simulink model "wheel_leg"  (R2024b)
settings: Solver=FixedStepAuto  StartTime=0.0  StopTime=10  FixedStep=0.001  RelTol=1e-3  AbsTol=1e-3  EnableMultiTasking=on
model workspace: external: MATLAB File UseBodyVel.m (data not in the file)
values from neighbouring files (symbols this model uses):
  g = 9.81    [LQR_calc.m]    (also in UseBodyVel.m)
  joint_distance = 0.11    [LQR_calc.m]    (also in UseBodyVel.m)
  l = -0.014    [LQR_calc.m]    (also in UseBodyVel.m)
  l_active_leg = 0.14    [LQR_calc.m]    (also in UseBodyVel.m)
  l_slave_leg = 0.24    [LQR_calc.m]    (also in UseBodyVel.m)
  M = 12    [LQR_calc.m]    (also in UseBodyVel.m)
  m_active_leg = 0.174    [LQR_calc.m]    (also in UseBodyVel.m)
  m_slave_leg = 0.180    (= 0.18)    [LQR_calc.m]    (also in UseBodyVel.m)
  mw = 0.58    [LQR_calc.m]    (also in UseBodyVel.m)
  N = mp*(x_ddot+L*theta_ddot*cos(theta)-L*theta_dot^2*sin(theta))+N_M    [UseBodyVel.m]
  X = [theta,theta_dot,x,x_dot,phi,phi_dot].'    [UseBodyVel.m]
undefined symbols (not defined in the file or in its folder): Y, Z
libraries: sm_lib x65, nesl_utility x25, dspfdesign x3
(part 3 of 3)

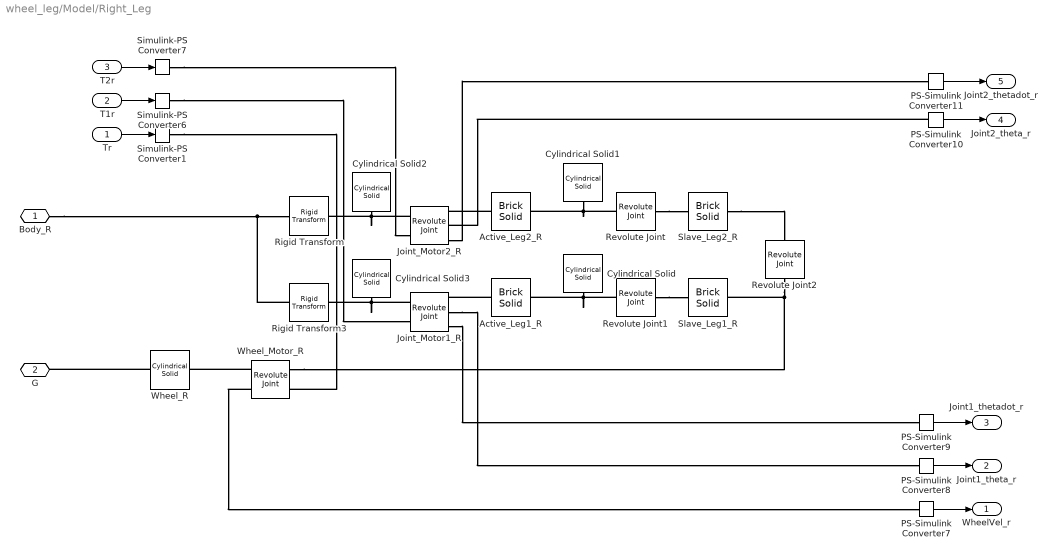
== system wheel_leg/Model/Right_Leg ==
  Tr : Inport
  T1r : Inport  Port=2
  T2r : Inport  Port=3
  Active_Leg1_R : sm_lib/Body Elements/Brick Solid  BrickDimensions=[0.02 l_active_leg 0.01]  BrickDimensionsUnits=m  ExportEntireGeometry=off  InertiaType=CalculateFromGeometry  BasedOnType=Mass  Density=1000  DensityUnits=kg/m^3  Mass=m_active_leg  MassUnits=kg  CenterOfMass=[0 0 0]  CenterOfMassUnits=m  MomentsOfInertia=[1 1 1]  MomentsOfInertiaUnits=kg*m^2  ProductsOfInertia=[0 0 0]  ProductsOfInertiaUnits=kg*m^2  GraphicType=FromGeometry  MarkerShape=Sphere  MarkerSize=10  GraphicVisPropType=SimpleVisualProperties  GraphicDiffuseColor=[0.5 0.5 0.5]  GraphicOpacity=1.0  GraphicSpecularColor=[0.5 0.5 0.5 1.0]  GraphicAmbientColor=[0.15 0.15 0.15 1.0]  GraphicEmissiveColor=[0.0 0.0 0.0 1.0]  GraphicShininess=75  DoExposeReferenceFrame=off  SerializedFrames=<Frames><Frame><Id>Frame1</Id><Value><Name>T</Name><Origin><Source>GeometricFeature</Source><FeatureName>+y surface</FeatureName></Origin><PrimaryAxis><DefinedDirection>+Z</DefinedDirection><Source>ReferenceFrame</Source><SourceDirection>+Z</SourceDirection><FeatureName></FeatureName></PrimaryAxis><SecondaryAxis><DefinedDirection>+X</DefinedDirection><Source>ReferenceFrame</Source><SourceDirection>+X</SourceDirection><FeatureName></FeatureName></SecondaryAxis></Value></Frame><Frame><Id>Frame2</Id><Value><Name>B</Name><Origin><Source>GeometricFeature</Source><FeatureName>-y surface</FeatureName></Origin><PrimaryAxis><DefinedDirection>+Z</DefinedDirection><Source>ReferenceFrame</Source><SourceDirection>+Z</SourceDirection><FeatureName></FeatureName></PrimaryAxis><SecondaryAxis><DefinedDirection>+X</DefinedDirection><Source>ReferenceFrame</Source><SourceDirection>+X</SourceDirection><FeatureName></FeatureName></SecondaryAxis></Value></Frame></Frames>
  Active_Leg2_R : sm_lib/Body Elements/Brick Solid  BrickDimensions=[0.02 l_active_leg 0.01]  BrickDimensionsUnits=m  ExportEntireGeometry=off  InertiaType=CalculateFromGeometry  BasedOnType=Mass  Density=1000  DensityUnits=kg/m^3  Mass=m_active_leg  MassUnits=kg  CenterOfMass=[0 0 0]  CenterOfMassUnits=m  MomentsOfInertia=[1 1 1]  MomentsOfInertiaUnits=kg*m^2  ProductsOfInertia=[0 0 0]  ProductsOfInertiaUnits=kg*m^2  GraphicType=FromGeometry  MarkerShape=Sphere  MarkerSize=10  GraphicVisPropType=SimpleVisualProperties  GraphicDiffuseColor=[0.5 0.5 0.5]  GraphicOpacity=1.0  GraphicSpecularColor=[0.5 0.5 0.5 1.0]  GraphicAmbientColor=[0.15 0.15 0.15 1.0]  GraphicEmissiveColor=[0.0 0.0 0.0 1.0]  GraphicShininess=75  DoExposeReferenceFrame=off  SerializedFrames=<Frames><Frame><Id>Frame1</Id><Value><Name>T</Name><Origin><Source>GeometricFeature</Source><FeatureName>+y surface</FeatureName></Origin><PrimaryAxis><DefinedDirection>+Z</DefinedDirection><Source>ReferenceFrame</Source><SourceDirection>+Z</SourceDirection><FeatureName></FeatureName></PrimaryAxis><SecondaryAxis><DefinedDirection>+X</DefinedDirection><Source>ReferenceFrame</Source><SourceDirection>+X</SourceDirection><FeatureName></FeatureName></SecondaryAxis></Value></Frame><Frame><Id>Frame2</Id><Value><Name>B</Name><Origin><Source>GeometricFeature</Source><FeatureName>-y surface</FeatureName></Origin><PrimaryAxis><DefinedDirection>+Z</DefinedDirection><Source>ReferenceFrame</Source><SourceDirection>+Z</SourceDirection><FeatureName></FeatureName></PrimaryAxis><SecondaryAxis><DefinedDirection>+X</DefinedDirection><Source>ReferenceFrame</Source><SourceDirection>+X</SourceDirection><FeatureName></FeatureName></SecondaryAxis></Value></Frame></Frames>
  Cylindrical Solid : sm_lib/Body Elements/Cylindrical Solid  CylinderRadius=0.01  CylinderRadiusUnits=m  CylinderLength=0.03  CylinderLengthUnits=m  ExportEntireGeometry=off  InertiaType=CalculateFromGeometry  BasedOnType=Mass  Density=1000  DensityUnits=kg/m^3  Mass=0  MassUnits=kg  CenterOfMass=[0 0 0]  CenterOfMassUnits=m  MomentsOfInertia=[1 1 1]  MomentsOfInertiaUnits=kg*m^2  ProductsOfInertia=[0 0 0]  ProductsOfInertiaUnits=kg*m^2  GraphicType=FromGeometry  MarkerShape=Sphere  MarkerSize=10  GraphicVisPropType=SimpleVisualProperties  GraphicDiffuseColor=[0 1 0]  GraphicOpacity=1.0  GraphicSpecularColor=[0.5 0.5 0.5 1.0]  GraphicAmbientColor=[0.15 0.15 0.15 1.0]  GraphicEmissiveColor=[0.0 0.0 0.0 1.0]  GraphicShininess=75  DoExposeReferenceFrame=on  SerializedFrames=<Frames/>
  Cylindrical Solid1 : sm_lib/Body Elements/Cylindrical Solid  CylinderRadius=0.01  CylinderRadiusUnits=m  CylinderLength=0.03  CylinderLengthUnits=m  ExportEntireGeometry=off  InertiaType=CalculateFromGeometry  BasedOnType=Mass  Density=1000  DensityUnits=kg/m^3  Mass=0  MassUnits=kg  CenterOfMass=[0 0 0]  CenterOfMassUnits=m  MomentsOfInertia=[1 1 1]  MomentsOfInertiaUnits=kg*m^2  ProductsOfInertia=[0 0 0]  ProductsOfInertiaUnits=kg*m^2  GraphicType=FromGeometry  MarkerShape=Sphere  MarkerSize=10  GraphicVisPropType=SimpleVisualProperties  GraphicDiffuseColor=[0 1 0]  GraphicOpacity=1.0  GraphicSpecularColor=[0.5 0.5 0.5 1.0]  GraphicAmbientColor=[0.15 0.15 0.15 1.0]  GraphicEmissiveColor=[0.0 0.0 0.0 1.0]  GraphicShininess=75  DoExposeReferenceFrame=on  SerializedFrames=<Frames/>
  Cylindrical Solid2 : sm_lib/Body Elements/Cylindrical Solid  CylinderRadius=0.02  CylinderRadiusUnits=m  CylinderLength=0.02  CylinderLengthUnits=m  ExportEntireGeometry=off  InertiaType=CalculateFromGeometry  BasedOnType=Mass  Density=1000  DensityUnits=kg/m^3  Mass=0  MassUnits=kg  CenterOfMass=[0 0 0]  CenterOfMassUnits=m  MomentsOfInertia=[1 1 1]  MomentsOfInertiaUnits=kg*m^2  ProductsOfInertia=[0 0 0]  ProductsOfInertiaUnits=kg*m^2  GraphicType=FromGeometry  MarkerShape=Sphere  MarkerSize=10  GraphicVisPropType=SimpleVisualProperties  GraphicDiffuseColor=[1.0 0.6 0.6]  GraphicOpacity=1.0  GraphicSpecularColor=[0.5 0.5 0.5 1.0]  GraphicAmbientColor=[0.15 0.15 0.15 1.0]  GraphicEmissiveColor=[0.0 0.0 0.0 1.0]  GraphicShininess=75  DoExposeReferenceFrame=on  SerializedFrames=<Frames/>
  Cylindrical Solid3 : sm_lib/Body Elements/Cylindrical Solid  CylinderRadius=0.02  CylinderRadiusUnits=m  CylinderLength=0.02  CylinderLengthUnits=m  ExportEntireGeometry=off  InertiaType=CalculateFromGeometry  BasedOnType=Mass  Density=1000  DensityUnits=kg/m^3  Mass=0  MassUnits=kg  CenterOfMass=[0 0 0]  CenterOfMassUnits=m  MomentsOfInertia=[1 1 1]  MomentsOfInertiaUnits=kg*m^2  ProductsOfInertia=[0 0 0]  ProductsOfInertiaUnits=kg*m^2  GraphicType=FromGeometry  MarkerShape=Sphere  MarkerSize=10  GraphicVisPropType=SimpleVisualProperties  GraphicDiffuseColor=[1.0 0.6 0.6]  GraphicOpacity=1.0  GraphicSpecularColor=[0.5 0.5 0.5 1.0]  GraphicAmbientColor=[0.15 0.15 0.15 1.0]  GraphicEmissiveColor=[0.0 0.0 0.0 1.0]  GraphicShininess=75  DoExposeReferenceFrame=on  SerializedFrames=<Frames/>
  Joint_Motor1_R : sm_lib/Joints/Revolute Joint  JointMode=Normal  CompositeWrenchDir=FollowerOnBase  CompositeWrenchFrame=BaseFrame  SenseConstraintForce=off  SenseConstraintTorque=off  SenseTotalForce=off  SenseTotalTorque=off  PositionTargetSpecify=on  PositionTargetPriority=High  PositionTargetValue=-50  PositionTargetValueUnits=deg  VelocityTargetSpecify=off  VelocityTargetPriority=High  VelocityTargetValue=0  VelocityTargetValueUnits=deg/s  EquilibriumPosition=0  EquilibriumPositionUnits=deg  SpringStiffness=0  SpringStiffnessUnits=N*m/deg  DampingCoefficient=0  DampingCoefficientUnits=N*m/(deg/s)  LowerLimitSpecify=off  LowerLimitBound=-100  LowerLimitBoundUnits=deg  LowerLimitStiffness=1e4  LowerLimitStiffnessUnits=N*m/deg  LowerLimitDamping=10  LowerLimitDampingUnits=N*m/(deg/s)  LowerLimitTransitionRegionWidth=0.1  LowerLimitTransitionRegionWidthUnits=deg  UpperLimitSpecify=off  UpperLimitBound=50  UpperLimitBoundUnits=deg  UpperLimitStiffness=1e4  UpperLimitStiffnessUnits=N*m/deg  UpperLimitDamping=10  UpperLimitDampingUnits=N*m/(deg/s)  UpperLimitTransitionRegionWidth=0.1  UpperLimitTransitionRegionWidthUnits=deg  TorqueActuationMode=InputTorque  MotionActuationMode=ComputedMotion  SensePosition=on  SenseVelocity=on  SenseAcceleration=off  SenseTorqueForce=off  SenseLowerLimitTorqueForce=off  SenseUpperLimitTorqueForce=off
  Joint_Motor2_R : sm_lib/Joints/Revolute Joint  JointMode=Normal  CompositeWrenchDir=FollowerOnBase  CompositeWrenchFrame=BaseFrame  SenseConstraintForce=off  SenseConstraintTorque=off  SenseTotalForce=off  SenseTotalTorque=off  PositionTargetSpecify=on  PositionTargetPriority=High  PositionTargetValue=50  PositionTargetValueUnits=deg  VelocityTargetSpecify=off  VelocityTargetPriority=High  VelocityTargetValue=0  VelocityTargetValueUnits=deg/s  EquilibriumPosition=0  EquilibriumPositionUnits=deg  SpringStiffness=0  SpringStiffnessUnits=N*m/deg  DampingCoefficient=0  DampingCoefficientUnits=N*m/(deg/s)  LowerLimitSpecify=off  LowerLimitBound=10  LowerLimitBoundUnits=deg  LowerLimitStiffness=1e4  LowerLimitStiffnessUnits=N*m/deg  LowerLimitDamping=10  LowerLimitDampingUnits=N*m/(deg/s)  LowerLimitTransitionRegionWidth=0.1  LowerLimitTransitionRegionWidthUnits=deg  UpperLimitSpecify=off  UpperLimitBound=100  UpperLimitBoundUnits=deg  UpperLimitStiffness=1e4  UpperLimitStiffnessUnits=N*m/deg  UpperLimitDamping=10  UpperLimitDampingUnits=N*m/(deg/s)  UpperLimitTransitionRegionWidth=0.1  UpperLimitTransitionRegionWidthUnits=deg  TorqueActuationMode=InputTorque  MotionActuationMode=ComputedMotion  SensePosition=on  SenseVelocity=on  SenseAcceleration=off  SenseTorqueForce=off  SenseLowerLimitTorqueForce=off  SenseUpperLimitTorqueForce=off
  PS-Simulink Converter10 : nesl_utility/PS-Simulink Converter  PhysicalDomain=network_engine_domain  SubClassName=ps_output  LeftPortType=input  RightPortType=output  PseudoPeriodic=off  Frequencies=[]  VectorFormat=inherit  Unit=rad  AffineConversion=off
  PS-Simulink Converter11 : nesl_utility/PS-Simulink Converter  PhysicalDomain=network_engine_domain  SubClassName=ps_output  LeftPortType=input  RightPortType=output  PseudoPeriodic=off  Frequencies=[]  VectorFormat=inherit  Unit=rad/s  AffineConversion=off
  PS-Simulink Converter7 : nesl_utility/PS-Simulink Converter  PhysicalDomain=network_engine_domain  SubClassName=ps_output  LeftPortType=input  RightPortType=output  PseudoPeriodic=off  Frequencies=[]  VectorFormat=inherit  Unit=rad/s  AffineConversion=off
  PS-Simulink Converter8 : nesl_utility/PS-Simulink Converter  PhysicalDomain=network_engine_domain  SubClassName=ps_output  LeftPortType=input  RightPortType=output  PseudoPeriodic=off  Frequencies=[]  VectorFormat=inherit  Unit=rad  AffineConversion=off
  PS-Simulink Converter9 : nesl_utility/PS-Simulink Converter  PhysicalDomain=network_engine_domain  SubClassName=ps_output  LeftPortType=input  RightPortType=output  PseudoPeriodic=off  Frequencies=[]  VectorFormat=inherit  Unit=rad/s  AffineConversion=off
  Revolute Joint : sm_lib/Joints/Revolute Joint  JointMode=Normal  CompositeWrenchDir=FollowerOnBase  CompositeWrenchFrame=BaseFrame  SenseConstraintForce=off  SenseConstraintTorque=off  SenseTotalForce=off  SenseTotalTorque=off  PositionTargetSpecify=off  PositionTargetPriority=High  PositionTargetValue=0  PositionTargetValueUnits=deg  VelocityTargetSpecify=off  VelocityTargetPriority=High  VelocityTargetValue=0  VelocityTargetValueUnits=deg/s  EquilibriumPosition=0  EquilibriumPositionUnits=deg  SpringStiffness=0  SpringStiffnessUnits=N*m/deg  DampingCoefficient=0  DampingCoefficientUnits=N*m/(deg/s)  LowerLimitSpecify=off  LowerLimitBound=-90  LowerLimitBoundUnits=deg  LowerLimitStiffness=1e4  LowerLimitStiffnessUnits=N*m/deg  LowerLimitDamping=10  LowerLimitDampingUnits=N*m/(deg/s)  LowerLimitTransitionRegionWidth=0.1  LowerLimitTransitionRegionWidthUnits=deg  UpperLimitSpecify=off  UpperLimitBound=90  UpperLimitBoundUnits=deg  UpperLimitStiffness=1e4  UpperLimitStiffnessUnits=N*m/deg  UpperLimitDamping=10  UpperLimitDampingUnits=N*m/(deg/s)  UpperLimitTransitionRegionWidth=0.1  UpperLimitTransitionRegionWidthUnits=deg  TorqueActuationMode=NoTorque  MotionActuationMode=ComputedMotion  SensePosition=off  SenseVelocity=off  SenseAcceleration=off  SenseTorqueForce=off  SenseLowerLimitTorqueForce=off  SenseUpperLimitTorqueForce=off
  Revolute Joint1 : sm_lib/Joints/Revolute Joint  JointMode=Normal  CompositeWrenchDir=FollowerOnBase  CompositeWrenchFrame=BaseFrame  SenseConstraintForce=off  SenseConstraintTorque=off  SenseTotalForce=off  SenseTotalTorque=off  PositionTargetSpecify=off  PositionTargetPriority=High  PositionTargetValue=0  PositionTargetValueUnits=deg  VelocityTargetSpecify=off  VelocityTargetPriority=High  VelocityTargetValue=0  VelocityTargetValueUnits=deg/s  EquilibriumPosition=0  EquilibriumPositionUnits=deg  SpringStiffness=0  SpringStiffnessUnits=N*m/deg  DampingCoefficient=0  DampingCoefficientUnits=N*m/(deg/s)  LowerLimitSpecify=off  LowerLimitBound=-90  LowerLimitBoundUnits=deg  LowerLimitStiffness=1e4  LowerLimitStiffnessUnits=N*m/deg  LowerLimitDamping=10  LowerLimitDampingUnits=N*m/(deg/s)  LowerLimitTransitionRegionWidth=0.1  LowerLimitTransitionRegionWidthUnits=deg  UpperLimitSpecify=off  UpperLimitBound=90  UpperLimitBoundUnits=deg  UpperLimitStiffness=1e4  UpperLimitStiffnessUnits=N*m/deg  UpperLimitDamping=10  UpperLimitDampingUnits=N*m/(deg/s)  UpperLimitTransitionRegionWidth=0.1  UpperLimitTransitionRegionWidthUnits=deg  TorqueActuationMode=NoTorque  MotionActuationMode=ComputedMotion  SensePosition=off  SenseVelocity=off  SenseAcceleration=off  SenseTorqueForce=off  SenseLowerLimitTorqueForce=off  SenseUpperLimitTorqueForce=off
  Revolute Joint2 : sm_lib/Joints/Revolute Joint  JointMode=Normal  CompositeWrenchDir=FollowerOnBase  CompositeWrenchFrame=BaseFrame  SenseConstraintForce=off  SenseConstraintTorque=off  SenseTotalForce=off  SenseTotalTorque=off  PositionTargetSpecify=off  PositionTargetPriority=High  PositionTargetValue=0  PositionTargetValueUnits=deg  VelocityTargetSpecify=off  VelocityTargetPriority=High  VelocityTargetValue=0  VelocityTargetValueUnits=deg/s  EquilibriumPosition=0  EquilibriumPositionUnits=deg  SpringStiffness=0  SpringStiffnessUnits=N*m/deg  DampingCoefficient=0  DampingCoefficientUnits=N*m/(deg/s)  LowerLimitSpecify=off  LowerLimitBound=-90  LowerLimitBoundUnits=deg  LowerLimitStiffness=1e4  LowerLimitStiffnessUnits=N*m/deg  LowerLimitDamping=10  LowerLimitDampingUnits=N*m/(deg/s)  LowerLimitTransitionRegionWidth=0.1  LowerLimitTransitionRegionWidthUnits=deg  UpperLimitSpecify=off  UpperLimitBound=90  UpperLimitBoundUnits=deg  UpperLimitStiffness=1e4  UpperLimitStiffnessUnits=N*m/deg  UpperLimitDamping=10  UpperLimitDampingUnits=N*m/(deg/s)  UpperLimitTransitionRegionWidth=0.1  UpperLimitTransitionRegionWidthUnits=deg  TorqueActuationMode=NoTorque  MotionActuationMode=ComputedMotion  SensePosition=off  SenseVelocity=off  SenseAcceleration=off  SenseTorqueForce=off  SenseLowerLimitTorqueForce=off  SenseUpperLimitTorqueForce=off
  Rigid Transform : sm_lib/Frames and Transforms/Rigid Transform  RotationMethod=None  FollAlignAxisA=+X  BaseAlignAxisA=+Y  FollAlignAxisB=+Y  BaseAlignAxisB=+Z  RotationStandardAxis=+Z  RotationAngle=0.0  RotationAngleUnits=deg  RotationArbitraryAxis=[0 0 1]  RotationSequenceAxes=FollowerAxes  RotationSequence=XYX  RotationSequenceAngles=[0 0 0]  RotationSequenceAnglesUnits=deg  RotationMatrix=[1 0 0; 0 1 0; 0 0 1]  Quaternion=[1 0 0 0]  TranslationMethod=Cartesian  TranslationCartesianOffset=[joint_distance/2 -l 0]  TranslationCartesianOffsetUnits=m  TranslationStandardAxis=+Z  TranslationStandardOffset=0  TranslationStandardOffsetUnits=m  TranslationROffset=0  TranslationROffsetUnits=m  TranslationThetaOffset=0  TranslationThetaOffsetUnits=deg  TranslationZOffset=0  TranslationZOffsetUnits=m
  Rigid Transform3 : sm_lib/Frames and Transforms/Rigid Transform  RotationMethod=None  FollAlignAxisA=+X  BaseAlignAxisA=+Y  FollAlignAxisB=+Y  BaseAlignAxisB=+Z  RotationStandardAxis=+Z  RotationAngle=0.0  RotationAngleUnits=deg  RotationArbitraryAxis=[0 0 1]  RotationSequenceAxes=FollowerAxes  RotationSequence=XYX  RotationSequenceAngles=[0 0 0]  RotationSequenceAnglesUnits=deg  RotationMatrix=[1 0 0; 0 1 0; 0 0 1]  Quaternion=[1 0 0 0]  TranslationMethod=Cartesian  TranslationCartesianOffset=[-joint_distance/2 -l 0]  TranslationCartesianOffsetUnits=m  TranslationStandardAxis=+Z  TranslationStandardOffset=0  TranslationStandardOffsetUnits=m  TranslationROffset=0  TranslationROffsetUnits=m  TranslationThetaOffset=0  TranslationThetaOffsetUnits=deg  TranslationZOffset=0  TranslationZOffsetUnits=m
  Simulink-PS Converter1 : nesl_utility/Simulink-PS Converter  PhysicalDomain=network_engine_domain  SubClassName=ps_input  LeftPortType=input  RightPortType=output  PseudoPeriodic=off  Frequencies=[]  NoiseDistribution=none  NoiseParameters=[]  Unit=N*m  AffineConversion=off  FilteringAndDerivatives=provide  SimscapeFilterOrder=1  InputFilterTimeConstant=0.001  UdotUserProvided=0
  Simulink-PS Converter6 : nesl_utility/Simulink-PS Converter  PhysicalDomain=network_engine_domain  SubClassName=ps_input  LeftPortType=input  RightPortType=output  PseudoPeriodic=off  Frequencies=[]  NoiseDistribution=none  NoiseParameters=[]  Unit=N*m  AffineConversion=off  FilteringAndDerivatives=provide  SimscapeFilterOrder=1  InputFilterTimeConstant=0.001  UdotUserProvided=0
  Simulink-PS Converter7 : nesl_utility/Simulink-PS Converter  PhysicalDomain=network_engine_domain  SubClassName=ps_input  LeftPortType=input  RightPortType=output  PseudoPeriodic=off  Frequencies=[]  NoiseDistribution=none  NoiseParameters=[]  Unit=N*m  AffineConversion=off  FilteringAndDerivatives=provide  SimscapeFilterOrder=1  InputFilterTimeConstant=0.001  UdotUserProvided=0
  Slave_Leg1_R : sm_lib/Body Elements/Brick Solid  BrickDimensions=[0.02 l_slave_leg 0.01]  BrickDimensionsUnits=m  ExportEntireGeometry=off  InertiaType=CalculateFromGeometry  BasedOnType=Mass  Density=1000  DensityUnits=kg/m^3  Mass=m_slave_leg  MassUnits=kg  CenterOfMass=[0 0 0]  CenterOfMassUnits=m  MomentsOfInertia=[1 1 1]  MomentsOfInertiaUnits=kg*m^2  ProductsOfInertia=[0 0 0]  ProductsOfInertiaUnits=kg*m^2  GraphicType=FromGeometry  MarkerShape=Sphere  MarkerSize=10  GraphicVisPropType=SimpleVisualProperties  GraphicDiffuseColor=[0.5 0.5 0.5]  GraphicOpacity=1.0  GraphicSpecularColor=[0.5 0.5 0.5 1.0]  GraphicAmbientColor=[0.15 0.15 0.15 1.0]  GraphicEmissiveColor=[0.0 0.0 0.0 1.0]  GraphicShininess=75  DoExposeReferenceFrame=off  SerializedFrames=<Frames><Frame><Id>Frame1</Id><Value><Name>T</Name><Origin><Source>GeometricFeature</Source><FeatureName>+y surface</FeatureName></Origin><PrimaryAxis><DefinedDirection>+Z</DefinedDirection><Source>ReferenceFrame</Source><SourceDirection>+Z</SourceDirection><FeatureName></FeatureName></PrimaryAxis><SecondaryAxis><DefinedDirection>+X</DefinedDirection><Source>ReferenceFrame</Source><SourceDirection>+X</SourceDirection><FeatureName></FeatureName></SecondaryAxis></Value></Frame><Frame><Id>Frame2</Id><Value><Name>B</Name><Origin><Source>GeometricFeature</Source><FeatureName>-y surface</FeatureName></Origin><PrimaryAxis><DefinedDirection>+Z</DefinedDirection><Source>ReferenceFrame</Source><SourceDirection>+Z</SourceDirection><FeatureName></FeatureName></PrimaryAxis><SecondaryAxis><DefinedDirection>+X</DefinedDirection><Source>ReferenceFrame</Source><SourceDirection>+X</SourceDirection><FeatureName></FeatureName></SecondaryAxis></Value></Frame></Frames>
  Slave_Leg2_R : sm_lib/Body Elements/Brick Solid  BrickDimensions=[0.02 l_slave_leg 0.01]  BrickDimensionsUnits=m  ExportEntireGeometry=off  InertiaType=CalculateFromGeometry  BasedOnType=Mass  Density=1000  DensityUnits=kg/m^3  Mass=m_slave_leg  MassUnits=kg  CenterOfMass=[0 0 0]  CenterOfMassUnits=m  MomentsOfInertia=[1 1 1]  MomentsOfInertiaUnits=kg*m^2  ProductsOfInertia=[0 0 0]  ProductsOfInertiaUnits=kg*m^2  GraphicType=FromGeometry  MarkerShape=Sphere  MarkerSize=10  GraphicVisPropType=SimpleVisualProperties  GraphicDiffuseColor=[0.5 0.5 0.5]  GraphicOpacity=1.0  GraphicSpecularColor=[0.5 0.5 0.5 1.0]  GraphicAmbientColor=[0.15 0.15 0.15 1.0]  GraphicEmissiveColor=[0.0 0.0 0.0 1.0]  GraphicShininess=75  DoExposeReferenceFrame=off  SerializedFrames=<Frames><Frame><Id>Frame1</Id><Value><Name>T</Name><Origin><Source>GeometricFeature</Source><FeatureName>+y surface</FeatureName></Origin><PrimaryAxis><DefinedDirection>+Z</DefinedDirection><Source>ReferenceFrame</Source><SourceDirection>+Z</SourceDirection><FeatureName></FeatureName></PrimaryAxis><SecondaryAxis><DefinedDirection>+X</DefinedDirection><Source>ReferenceFrame</Source><SourceDirection>+X</SourceDirection><FeatureName></FeatureName></SecondaryAxis></Value></Frame><Frame><Id>Frame2</Id><Value><Name>B</Name><Origin><Source>GeometricFeature</Source><FeatureName>-y surface</FeatureName></Origin><PrimaryAxis><DefinedDirection>+Z</DefinedDirection><Source>ReferenceFrame</Source><SourceDirection>+Z</SourceDirection><FeatureName></FeatureName></PrimaryAxis><SecondaryAxis><DefinedDirection>+X</DefinedDirection><Source>ReferenceFrame</Source><SourceDirection>+X</SourceDirection><FeatureName></FeatureName></SecondaryAxis></Value></Frame></Frames>
  Wheel_Motor_R : sm_lib/Joints/Revolute Joint  JointMode=Normal  CompositeWrenchDir=FollowerOnBase  CompositeWrenchFrame=BaseFrame  SenseConstraintForce=off  SenseConstraintTorque=off  SenseTotalForce=off  SenseTotalTorque=off  PositionTargetSpecify=off  PositionTargetPriority=High  PositionTargetValue=0  PositionTargetValueUnits=deg  VelocityTargetSpecify=off  VelocityTargetPriority=High  VelocityTargetValue=0  VelocityTargetValueUnits=deg/s  EquilibriumPosition=0  EquilibriumPositionUnits=deg  SpringStiffness=0  SpringStiffnessUnits=N*m/deg  DampingCoefficient=0  DampingCoefficientUnits=N*m/(deg/s)  LowerLimitSpecify=off  LowerLimitBound=-90  LowerLimitBoundUnits=deg  LowerLimitStiffness=1e4  LowerLimitStiffnessUnits=N*m/deg  LowerLimitDamping=10  LowerLimitDampingUnits=N*m/(deg/s)  LowerLimitTransitionRegionWidth=0.1  LowerLimitTransitionRegionWidthUnits=deg  UpperLimitSpecify=off  UpperLimitBound=90  UpperLimitBoundUnits=deg  UpperLimitStiffness=1e4  UpperLimitStiffnessUnits=N*m/deg  UpperLimitDamping=10  UpperLimitDampingUnits=N*m/(deg/s)  UpperLimitTransitionRegionWidth=0.1  UpperLimitTransitionRegionWidthUnits=deg  TorqueActuationMode=InputTorque  MotionActuationMode=ComputedMotion  SensePosition=off  SenseVelocity=on  SenseAcceleration=off  SenseTorqueForce=off  SenseLowerLimitTorqueForce=off  SenseUpperLimitTorqueForce=off
  Wheel_R : sm_lib/Body Elements/Cylindrical Solid  CylinderRadius=R  CylinderRadiusUnits=m  CylinderLength=0.03  CylinderLengthUnits=m  ExportEntireGeometry=on  InertiaType=CalculateFromGeometry  BasedOnType=Mass  Density=1000  DensityUnits=kg/m^3  Mass=mw  MassUnits=kg  CenterOfMass=[0 0 0]  CenterOfMassUnits=m  MomentsOfInertia=[1 1 1]  MomentsOfInertiaUnits=kg*m^2  ProductsOfInertia=[0 0 0]  ProductsOfInertiaUnits=kg*m^2  GraphicType=FromGeometry  MarkerShape=Sphere  MarkerSize=10  GraphicVisPropType=SimpleVisualProperties  GraphicDiffuseColor=[1.0 0.2 0.2]  GraphicOpacity=1.0  GraphicSpecularColor=[0.5 0.5 0.5 1.0]  GraphicAmbientColor=[0.15 0.15 0.15 1.0]  GraphicEmissiveColor=[0.0 0.0 0.0 1.0]  GraphicShininess=75  DoExposeReferenceFrame=on  SerializedFrames=<Frames/>
  Body_R : PMIOPort  Side=Left
  G : PMIOPort  Port=2  Side=Left
  WheelVel_r : Outport
  Joint1_theta_r : Outport  Port=2
  Joint1_thetadot_r : Outport  Port=3
  Joint2_theta_r : Outport  Port=4
  Joint2_thetadot_r : Outport  Port=5
  wires:
  PS-Simulink Converter9/1 -> Joint1_thetadot_r/1
  T2r/1 -> Simulink-PS Converter7/1
  PS-Simulink Converter10/1 -> Joint2_theta_r/1
  PS-Simulink Converter11/1 -> Joint2_thetadot_r/1
  Tr/1 -> Simulink-PS Converter1/1
  T1r/1 -> Simulink-PS Converter6/1
  PS-Simulink Converter7/1 -> WheelVel_r/1
  PS-Simulink Converter8/1 -> Joint1_theta_r/1
  connections:
  Joint_Motor2_R/RConn3 -- PS-Simulink Converter11/LConn1
  Revolute Joint/LConn1 -- Cylindrical Solid1/RConn1 -- Active_Leg2_R/RConn1
  Rigid Transform3/LConn1 -- Body_R/RConn1 -- Rigid Transform/LConn1
  Revolute Joint/RConn1 -- Slave_Leg2_R/LConn1
  Slave_Leg2_R/RConn1 -- Revolute Joint2/LConn1
  Joint_Motor2_R/LConn1 -- Cylindrical Solid2/RConn1 -- Rigid Transform/RConn1
  Revolute Joint1/RConn1 -- Slave_Leg1_R/LConn1
  Revolute Joint2/RConn1 -- Wheel_Motor_R/LConn1 -- Slave_Leg1_R/RConn1
  Active_Leg2_R/LConn1 -- Joint_Motor2_R/RConn1
  Joint_Motor1_R/RConn3 -- PS-Simulink Converter9/LConn1
  Simulink-PS Converter6/RConn1 -- Joint_Motor1_R/LConn2
  Wheel_Motor_R/RConn1 -- Wheel_R/RConn1
  Active_Leg1_R/LConn1 -- Joint_Motor1_R/RConn1
  Revolute Joint1/LConn1 -- Cylindrical Solid/RConn1 -- Active_Leg1_R/RConn1
  Simulink-PS Converter7/RConn1 -- Joint_Motor2_R/LConn2
  PS-Simulink Converter10/LConn1 -- Joint_Motor2_R/RConn2
  Joint_Motor1_R/LConn1 -- Cylindrical Solid3/RConn1 -- Rigid Transform3/RConn1
  Wheel_Motor_R/RConn2 -- PS-Simulink Converter7/LConn1
  Joint_Motor1_R/RConn2 -- PS-Simulink Converter8/LConn1
  Simulink-PS Converter1/RConn1 -- Wheel_Motor_R/LConn2
  Wheel_R/LConn1 -- G/RConn1

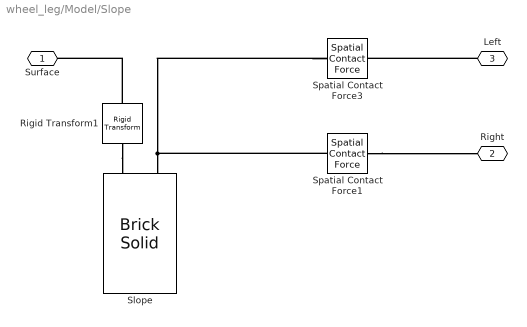
== system wheel_leg/Model/Slope ==
  Rigid Transform1 : sm_lib/Frames and Transforms/Rigid Transform  RotationMethod=StandardAxis  FollAlignAxisA=+X  BaseAlignAxisA=+Y  FollAlignAxisB=+Y  BaseAlignAxisB=+Z  RotationStandardAxis=+Z  RotationAngle=gradient  RotationAngleUnits=deg  RotationArbitraryAxis=[0 0 1]  RotationSequenceAxes=FollowerAxes  RotationSequence=XYX  RotationSequenceAngles=[0 0 0]  RotationSequenceAnglesUnits=deg  RotationMatrix=[1 0 0; 0 1 0; 0 0 1]  Quaternion=[1 0 0 0]  TranslationMethod=Cartesian  TranslationCartesianOffset=[8 0 0]  TranslationCartesianOffsetUnits=m  TranslationStandardAxis=+X  TranslationStandardOffset=5  TranslationStandardOffsetUnits=m  TranslationROffset=0  TranslationROffsetUnits=m  TranslationThetaOffset=0  TranslationThetaOffsetUnits=deg  TranslationZOffset=0  TranslationZOffsetUnits=m
  Slope : sm_lib/Body Elements/Brick Solid  BrickDimensions=[length 0.01 10]  BrickDimensionsUnits=m  ExportEntireGeometry=on  InertiaType=CalculateFromGeometry  BasedOnType=Density  Density=1000  DensityUnits=kg/m^3  Mass=1  MassUnits=kg  CenterOfMass=[0 0 0]  CenterOfMassUnits=m  MomentsOfInertia=[1 1 1]  MomentsOfInertiaUnits=kg*m^2  ProductsOfInertia=[0 0 0]  ProductsOfInertiaUnits=kg*m^2  GraphicType=FromGeometry  MarkerShape=Sphere  MarkerSize=10  GraphicVisPropType=SimpleVisualProperties  GraphicDiffuseColor=[1.0 0.4 1.0]  GraphicOpacity=1.0  GraphicSpecularColor=[0.5 0.5 0.5 1.0]  GraphicAmbientColor=[0.15 0.15 0.15 1.0]  GraphicEmissiveColor=[0.0 0.0 0.0 1.0]  GraphicShininess=75  DoExposeReferenceFrame=off  SerializedFrames=<Frames><Frame><Id>Frame2</Id><Value><Name>eage_B</Name><Origin><Source>GeometricFeature</Source><FeatureName>-x +y curve</FeatureName></Origin><PrimaryAxis><DefinedDirection>+Z</DefinedDirection><Source>ReferenceFrame</Source><SourceDirection>+Z</SourceDirection><FeatureName></FeatureName></PrimaryAxis><SecondaryAxis><DefinedDirection>+X</DefinedDirection><Source>ReferenceFrame</Source><SourceDirection>+X</SourceDirection><FeatureName></FeatureName></SecondaryAxis></Value></Frame><Frame><Id>Frame3</Id><Value><Name>eage_T</Name><Origin><Source>GeometricFeature</Source><FeatureName>+x +y curve</FeatureName></Origin><PrimaryAxis><DefinedDirection>+Z</DefinedDirection><Source>ReferenceFrame</Source><SourceDirection>+Z</SourceDirection><FeatureName></FeatureName></PrimaryAxis><SecondaryAxis><DefinedDirection>+X</DefinedDirection><Source>ReferenceFrame</Source><SourceDirection>+X</SourceDirection><FeatureName></FeatureName></SecondaryAxis></Value></Frame></Frames>
  Spatial Contact Force1 : sm_lib/Forces and Torques/Spatial Contact Force  NormalForceType=SmoothSpringDamper  NormalStiffness=1e6  NormalStiffnessUnits=N/m  NormalDamping=1e3  NormalDampingUnits=N/(m/s)  NormalTransitionRegionWidth=1e-4  NormalTransitionRegionWidthUnits=m  FrictionType=SmoothStickSlip  CoefficientOfStaticFriction=0.5  CoefficientOfDynamicFriction=0.3  FrictionalCriticalVelocity=1e-3  FrictionalCriticalVelocityUnits=m/s  SenseContactSignal=off  SensePenetrationDepth=off  SenseSeparationDistance=off  SenseNormalForceMagnitude=off  SenseFrictionalForceMagnitude=off  SenseNormalVelocity=off  SenseTangentialVelocity=off  SenseContactBaseRotation=off  SenseContactBaseTranslation=off  SenseContactFollowerRotation=off  SenseContactFollowerTranslation=off  ZeroCrossDetectContactStartAndEnd=off
  Spatial Contact Force3 : sm_lib/Forces and Torques/Spatial Contact Force  NormalForceType=SmoothSpringDamper  NormalStiffness=1e6  NormalStiffnessUnits=N/m  NormalDamping=1e3  NormalDampingUnits=N/(m/s)  NormalTransitionRegionWidth=1e-4  NormalTransitionRegionWidthUnits=m  FrictionType=SmoothStickSlip  CoefficientOfStaticFriction=0.5  CoefficientOfDynamicFriction=0.3  FrictionalCriticalVelocity=1e-3  FrictionalCriticalVelocityUnits=m/s  SenseContactSignal=off  SensePenetrationDepth=off  SenseSeparationDistance=off  SenseNormalForceMagnitude=off  SenseFrictionalForceMagnitude=off  SenseNormalVelocity=off  SenseTangentialVelocity=off  SenseContactBaseRotation=off  SenseContactBaseTranslation=off  SenseContactFollowerRotation=off  SenseContactFollowerTranslation=off  ZeroCrossDetectContactStartAndEnd=off
  Surface : PMIOPort  Side=Left
  Right : PMIOPort  Port=2  Side=Left
  Left : PMIOPort  Port=3  Side=Left
  connections:
  Rigid Transform1/RConn1 -- Slope/LConn1
  Spatial Contact Force1/LConn1 -- Spatial Contact Force3/LConn1 -- Slope/LConn2
  Spatial Contact Force1/RConn1 -- Right/RConn1
  Rigid Transform1/LConn1 -- Surface/RConn1
  Left/RConn1 -- Spatial Contact Force3/RConn1

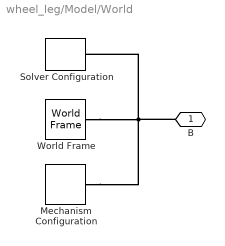
== system wheel_leg/Model/World ==
  Mechanism Configuration : sm_lib/Utilities/Mechanism Configuration  UniformGravity=Constant  GravityVector=[0 -g 0]  GravityVectorUnits=m/s^2  LinearizationDelta=0.001  JointModeTransitionNonlinearIterations=2
  Solver Configuration : nesl_utility/Solver Configuration  PhysicalDomain=network_engine_domain  SubClassName=solver  LeftPortType=input  RightPortType=generic  Tones=[]  Harmonics=[]  SimulateNoise=off  Profile=off  UseLocalSampling=off  EnableSwitchedLinearOptims=on  FrequencyDomain=off  UseCCode=off  RelTol=0.001  AbsTol=1e-06  MinStep=1e-09  ToWorkspace=off  RevertToSquareIcSolve=off  NumHomotopyIterations=100  PhasorMode=off  PhasorModeNumHarmonics=1  ConsistencySolver=NEWTON_XTOL_AFTER_FTOL  IndexReductionMethod=DerivativeReplacement  DoDC=off  ResidualTolerance=1e-09  ConsistencyTolSource=GLOBAL  ConsistencyAbsTol=0.001  ConsistencyRelTol=0.001  ConsistencyTolFactor=0.001  UseLocalSolver=off  LocalSolverChoice=NE_BACKWARD_EULER_ADVANCER  ResolveIndetEquations=on  FunctionEvalNumThread=1  LocalSolverSampleTime=0.001  DoFixedCost=off  MaxNonlinIter=3  MaxModeIter=2  ComputeImpulses=off  ImpulseIterations=2  LinearAlgebra=Sparse  LinearAlgebraNumThread=0  EquationFormulation=NE_TIME_EF  DelaysMemoryBudget=1024  AutomaticFiltering=off  FilteringTimeConstant=0.001  PartitionStorageMethod=AS_NEEDED  PartitionMemoryBudget=1024  PartitionMethod=FAST  MultibodyUseLocalSolver=off  MultibodyLocalSolverChoice=ODE1  MultibodyLocalSolverSampleTime=0.001
  World Frame : sm_lib/Frames and Transforms/World Frame
  B : PMIOPort  Side=Right
  connections:
  World Frame/RConn1 -- B/RConn1 -- Solver Configuration/RConn1 -- Mechanism Configuration/RConn1

== matlab function wheel_leg/Model/MATLAB Function ==
  data: Yaw output; quat input; Pitch output; Roll output
function [Yaw,Pitch,Roll] = Quat_To_Euler(quat)

    % Rearrange the quaternion into the correct form [w, x, y, z]
    Quat = [quat(1,1), quat(2,1), quat(3,1), quat(4,1)];

    % Convert the quaternion to Euler angles using 'XYZ' order
    Euler = quat2eul(Quat, 'XYZ');

    % Extract the roll, pitch, and yaw angles from the Euler angles
    Roll = Euler(1);
    Yaw =Euler(2);
    Pitch = Euler(3);

end

== matlab function wheel_leg/SpeedEstimation/MATLAB Function4 ==
  settings: updateMethod=DISCRETE  sampleTime=0.001
  data: body_vr input; body_vl input; x_dot output; accx input; vel data_store_memory; vel_cov data_store_memory; accy input; pitch input
function x_dot = SpeedEstimation(body_vr, body_vl, accx, accy, pitch)

%% 变量及参数
global vel;             % 机体速度
global vel_cov;         % 速度协方差
PROCESS_NOISE = 1;   % 过程噪声
MEASURE_NOISE = 10000;   % 测量噪声
delta_t = 0.001;

%% 机体平动
vel_m = (body_vr + body_vl)/2;              % 速度测量值
acc_m = accx*cos(pitch) - accy*sin(pitch);  % 加速度测量值

%% 融合加速度计和机体速度
prior = vel + acc_m*delta_t;       % 先验估计值
cov = vel_cov + PROCESS_NOISE*delta_t;     % 先验协方差
k = cov/(cov + MEASURE_NOISE);     % 卡尔曼增益
vel = prior + k*(vel_m-prior);     % 后验估计值
vel_cov = cov*(1-k);               % 后验协方差

x_dot = vel;

%% 协方差限幅
if vel_cov > 100
    vel_cov = 100;
elseif vel_cov < 0.01
    vel_cov = 0.01;
end

end

== matlab function wheel_leg/Controller/MATLAB Function ==
  settings: updateMethod=DISCRETE
  data: x input; x_dot input; T output; pitch input; pitch_dot input; Joint1_theta input; Joint1_thetadot input; Joint2_theta input; Joint2_thetadot input; LegLength_ref input; x_ref input; T1 output; T2 output; Height output; x_dot_ref input; accx input; accy input; theta_dot_rlast data_store_memory; LegLength_dot_rlast data_store_memory; FN_r data_store_memory; FN output; l_active_leg data_store_memory; l_slave_leg data_store_memory; joint_distance data_store_memory; mw data_store_memory; g data_store_memory; K_cons data_store_memory; R data_store_memory; body_v output; WheelVel input
function [T,T1,T2,Height,FN,body_v]= Right_Leg(x,x_dot,pitch,pitch_dot,Joint1_theta,Joint1_thetadot,Joint2_theta,Joint2_thetadot,LegLength_ref,x_ref,x_dot_ref,accx,accy,WheelVel)
    
phi1 = -Joint1_theta + pi/2;
phi1_dot = -Joint1_thetadot;
phi4 = pi/2 -Joint2_theta;
phi4_dot = -Joint2_thetadot;

%% 全局变量
% global theta_dot_rlast;
% global LegLength_dot_rlast;
global FN_r;
global l_active_leg;
global l_slave_leg;
global joint_distance;
global mw;
global g;
global K_cons;
global R;

%% 结构参数
l1 = l_active_leg;
l4 = l_active_leg;
l2 = l_slave_leg;
l3 = l_slave_leg;
l5 = joint_distance;

%% 正运动学解算
xD = l5 + l4*cos(phi4);
yD = l4*sin(phi4);
xB = 0 + l1*cos(phi1);
yB = l1*sin(phi1);

BD = sqrt((xD-xB)^2+(yD-yB)^2); 
A0 = 2*l2*(xD-xB);
B0 = 2*l2*(yD-yB);
C0 = l2^2 + BD^2 - l3^2;
phi2 = 2*atan2(B0 + sqrt(A0^2+B0^2-C0^2),A0+C0);
xC = l1*cos(phi1) + l2*cos(phi2);
yC = l1*sin(phi1) + l2*sin(phi2);
phi3 = atan2(yC-yD,xC-xD);   % 稍后用于计算VMC

% theta and LegLength solve
phi5 = atan2(yC, xC-l5/2);
alpha = phi5 - pi/2;
theta = alpha - pitch;
LegLength = sqrt((xC-l5/2)^2+yC^2);
Height = LegLength*cos(theta);

%% 预测下一时刻
dt = 0.0001;
phi1_pre = phi1 + phi1_dot*dt;   
phi4_pre = phi4 + phi4_dot*dt;

% 重新计算腿长和角度
xD = l5 + l4*cos(phi4_pre);
yD = l4*sin(phi4_pre);
xB = 0 + l1*cos(phi1_pre);
yB = l1*sin(phi1_pre);

BD = sqrt((xD-xB)^2+(yD-yB)^2); 
A0 = 2*l2*(xD-xB);
B0 = 2*l2*(yD-yB);
C0 = l2^2 + BD^2 - l3^2;
phi2_pre = 2*atan2(B0 + sqrt(A0^2+B0^2-C0^2),A0+C0);
xC = l1*cos(phi1_pre) + l2*cos(phi2_pre);
yC = l1*sin(phi1_pre) + l2*sin(phi2_pre);

% theta_dot and LegLength solve
phi5_pre = atan2(yC, xC-l5/2);
phi2_dot = (phi2_pre-phi2)/dt;
theta_dot = (phi5_pre - pi/2 - (pitch+pitch_dot*dt) - theta)/dt;
LegLength_dot = (sqrt((xC-l5/2)^2+yC^2) - LegLength)/dt;
Height_dot = LegLength_dot*cos(theta) - LegLength*sin(theta)*theta_dot;


%% LQR_cal
% K多项式拟合
ll = [LegLength^2; LegLength; 1];
kk = K_cons*ll;

% 离地检测
if FN_r<20
    K_mat = [0 0 0 0 0 0;
            kk(7) kk(8) 0 0 0 0];
else
    K_mat = [kk(1) kk(2) kk(3) kk(4) kk(5) kk(6);
            kk(7) kk(8) kk(9) kk(10) kk(11) kk(12)];
end


% T T_leg solve
X_ref = [0 0 x_ref x_dot_ref 0 0]';
X = [theta theta_dot x x_dot pitch pitch_dot]';

X_err = X_ref - X;
u = K_mat*X_err;

T = -u(1);
T_Leg = u(2);


%% LegLength Control
Kp = 1200;
Kd = 300;
F_Leg = Kp*(LegLength_ref-Height) + Kd*(0-Height_dot);


%% T1 and T2 solve
F = [F_Leg; T_Leg];
Trans_Jacobian = [l1*sin(phi5-phi3)*sin(phi1-phi2)/sin(phi3-phi2)   l1*cos(phi5-phi3)*sin(phi1-phi2)/LegLength/sin(phi3-phi2);
                  l4*sin(phi5-phi2)*sin(phi3-phi4)/sin(phi3-phi2)   l4*cos(phi5-phi2)*sin(phi3-phi4)/LegLength/sin(phi3-phi2)];
Tj = Trans_Jacobian*F;

T1 = -Tj(1);
T2 = -Tj(2);


%% 驱动轮支持力解算
% delta = 0.01;
% theta_ddot = (theta_dot-theta_dot_rlast)/delta;
% leglen_ddot = (LegLength_dot-LegLength_dot_rlast)/delta;
% theta_dot_rlast = theta_dot;
% LegLength_dot_rlast = LegLength_dot;

yM_ddot = accx*sin(pitch) + accy*cos(pitch);
% yw_ddot = yM_ddot - leglen_ddot*cos(theta) + 2*LegLength_dot*theta_dot*sin(theta) + LegLength*theta_ddot*sin(theta) + LegLength*theta_dot^2*cos(theta);

P = F_Leg*cos(theta) + T_Leg*sin(theta)/LegLength;
FN_r = mw*yM_ddot + P + mw*g;
FN = FN_r;

%% 轮速修正
wheel_w = -WheelVel + phi2_dot - pitch_dot;

% 计算髋关节处速度
body_v = wheel_w*R + LegLength*theta_dot + LegLength_dot*sin(theta);

end

== matlab function wheel_leg/Controller/MATLAB Function1 ==
  settings: updateMethod=DISCRETE
  data: x input; x_dot input; T output; pitch input; pitch_dot input; Joint1_theta input; Joint1_thetadot input; Joint2_theta input; Joint2_thetadot input; LegLength_ref input; x_ref input; T1 output; T2 output; Height output; x_dot_ref input; accx input; accy input; theta_dot_llast data_store_memory; LegLength_dot_llast data_store_memory; FN_l data_store_memory; FN output; l_active_leg data_store_memory; l_slave_leg data_store_memory; mw data_store_memory; g data_store_memory; joint_distance data_store_memory; K_cons data_store_memory; WheelVel input; body_v output; R data_store_memory
function [T,T1,T2,Height,FN,body_v]= Left_Leg(x,x_dot,pitch,pitch_dot,Joint1_theta,Joint1_thetadot,Joint2_theta,Joint2_thetadot,LegLength_ref,x_ref,x_dot_ref,accx,accy,WheelVel)
    
phi1 = -Joint1_theta + pi/2;
phi1_dot = -Joint1_thetadot;
phi4 = pi/2 -Joint2_theta;
phi4_dot = -Joint2_thetadot;

%% 全局变量
% global theta_dot_llast;
% global LegLength_dot_llast;
global FN_l;
global l_active_leg;
global l_slave_leg;
global joint_distance;
global mw;
global g;
global K_cons;
global R;

%% 结构参数
l1 = l_active_leg;
l4 = l_active_leg;
l2 = l_slave_leg;
l3 = l_slave_leg;
l5 = joint_distance;

%% 正运动学解算
xD = l5 + l4*cos(phi4);
yD = l4*sin(phi4);
xB = 0 + l1*cos(phi1);
yB = l1*sin(phi1);

BD = sqrt((xD-xB)^2+(yD-yB)^2); 
A0 = 2*l2*(xD-xB);
B0 = 2*l2*(yD-yB);
C0 = l2^2 + BD^2 - l3^2;
phi2 = 2*atan2(B0 + sqrt(A0^2+B0^2-C0^2),A0+C0);
xC = l1*cos(phi1) + l2*cos(phi2);
yC = l1*sin(phi1) + l2*sin(phi2);
phi3 = atan2(yC-yD,xC-xD);   % 稍后用于计算VMC

% theta and LegLength solve
phi5 = atan2(yC, xC-l5/2);
alpha = phi5 - pi/2;
theta = alpha - pitch;
LegLength = sqrt((xC-l5/2)^2+yC^2);
Height = LegLength*cos(theta);

%% 预测下一时刻
dt = 0.0001;
phi1_pre = phi1 + phi1_dot*dt;   
phi4_pre = phi4 + phi4_dot*dt;

% 重新计算腿长和角度
xD = l5 + l4*cos(phi4_pre);
yD = l4*sin(phi4_pre);
xB = 0 + l1*cos(phi1_pre);
yB = l1*sin(phi1_pre);

BD = sqrt((xD-xB)^2+(yD-yB)^2); 
A0 = 2*l2*(xD-xB);
B0 = 2*l2*(yD-yB);
C0 = l2^2 + BD^2 - l3^2;
phi2_pre = 2*atan2(B0 + sqrt(A0^2+B0^2-C0^2),A0+C0);
xC = l1*cos(phi1_pre) + l2*cos(phi2_pre);
yC = l1*sin(phi1_pre) + l2*sin(phi2_pre);

% theta_dot and LegLength solve
phi5_pre = atan2(yC, xC-l5/2);
phi2_dot = (phi2_pre-phi2)/dt;
theta_dot = (phi5_pre - pi/2 - (pitch+pitch_dot*dt) - theta)/dt;
LegLength_dot = (sqrt((xC-l5/2)^2+yC^2) - LegLength)/dt;
Height_dot = LegLength_dot*cos(theta) - LegLength*sin(theta)*theta_dot;


%% LQR_cal
% K多项式拟合
ll = [LegLength^2; LegLength; 1];
kk = K_cons*ll;

% 离地检测
if FN_l<20
    K_mat = [0 0 0 0 0 0;
            kk(7) kk(8) 0 0 0 0];
else
    K_mat = [kk(1) kk(2) kk(3) kk(4) kk(5) kk(6);
            kk(7) kk(8) kk(9) kk(10) kk(11) kk(12)];
end

% T T_leg solve
X_ref = [0 0 x_ref x_dot_ref 0 0]';
X = [theta theta_dot x x_dot pitch pitch_dot]';

X_err = X_ref - X;
u = K_mat*X_err;

T = -u(1);
T_Leg = u(2);


%% LegLength Control
Kp = 1200;
Kd = 300;
F_Leg = Kp*(LegLength_ref-Height) + Kd*(0-Height_dot);


%% T1 and T2 solve
F = [F_Leg; T_Leg];
Trans_Jacobian = [l1*sin(phi5-phi3)*sin(phi1-phi2)/sin(phi3-phi2)   l1*cos(phi5-phi3)*sin(phi1-phi2)/LegLength/sin(phi3-phi2);
                  l4*sin(phi5-phi2)*sin(phi3-phi4)/sin(phi3-phi2)   l4*cos(phi5-phi2)*sin(phi3-phi4)/LegLength/sin(phi3-phi2)];
Tj = Trans_Jacobian*F;

T1 = -Tj(1);
T2 = -Tj(2);


%% 驱动轮支持力解算
% delta = 0.01;
% theta_ddot = (theta_dot-theta_dot_llast)/delta;
% leglen_ddot = (LegLength_dot-LegLength_dot_llast)/delta;
% theta_dot_llast = theta_dot;
% LegLength_dot_llast = LegLength_dot;

yM_ddot = accx*sin(pitch) + accy*cos(pitch);
% yw_ddot = yM_ddot - leglen_ddot*cos(theta) + 2*LegLength_dot*theta_dot*sin(theta) + LegLength*theta_ddot*sin(theta) + LegLength*theta_dot^2*cos(theta);

P = F_Leg*cos(theta) + T_Leg*sin(theta)/LegLength;
FN_l = mw*yM_ddot + P + mw*g;
FN = FN_l;

%% 轮速修正
wheel_w = -WheelVel + phi2_dot - pitch_dot;

% 计算髋关节处速度
body_v = wheel_w*R + LegLength*theta_dot + LegLength_dot*sin(theta);


end
